simulink model "Alpha_Drone_Model"  (R2020b)
settings: Solver=VariableStepAuto  StartTime=0.0  StopTime=5  RelTol=1e-3
model workspace (MATLAB code in the model file):
  | % -------------------------------------------------------------------
  | %  Generated by MATLAB on 1-Mar-2021 14:46:59
  | %  MATLAB version: 9.9.0.1495850 (R2020b) Update 1
  | % -------------------------------------------------------------------
  | 
  | 
  | smiData = struct;
  | smiData.RigidTransform = struct;
  | smiData.RigidTransform(1).translation = ...
  |   [0 0 0];
  | smiData.RigidTransform(1).angle = 3.1415926535897931;
  | smiData.RigidTransform(1).axis = [1 0 0];
  | smiData.RigidTransform(1).ID = ['B[drone_base_test_3-1:-:drone_camera_w' ...
  |                                 'all_test-1]'];
  | smiData.RigidTransform(2).translation = ...
  |   [88.000000000000028 19.999999999999986 6.00000000000003];
  | smiData.RigidTransform(2).angle = 2.0943951023931953;
  | smiData.RigidTransform(2).axis = [0.57735026918962584 0.57735026918962584 ...
  |                                   -0.57735026918962562];
  | smiData.RigidTransform(2).ID = ['F[drone_base_test_3-1:-:drone_camera_w' ...
  |                                 'all_test-1]'];
  | smiData.RigidTransform(3).translation = ...
  |   [0 0 0];
  | smiData.RigidTransform(3).angle = 3.1415926535897931;
  | smiData.RigidTransform(3).axis = [1 0 0];
  | smiData.RigidTransform(3).ID = ['B[drone_base_test_3-1:-:drone_camera_w' ...
  |                                 'all_test-2]'];
  | smiData.RigidTransform(4).translation = ...
  |   [87.999999999999858 19.999999999999854 26.999999999999904];
  | smiData.RigidTransform(4).angle = 2.0943951023931953;
  | smiData.RigidTransform(4).axis = [0.57735026918962373 0.57735026918962573 ...
  |                                   -0.57735026918962784];
  | smiData.RigidTransform(4).ID = ['F[drone_base_test_3-1:-:drone_camera_w' ...
  |                                 'all_test-2]'];
  | smiData.RigidTransform(5).translation = ...
  |   [30.733125881400653 59.62221317792671 4.0000000000000036];
  | smiData.RigidTransform(5).angle = 3.1415926535897931;
  | smiData.RigidTransform(5).axis = [1 0 0];
  | smiData.RigidTransform(5).ID = ['B[drone_base_test_3-1:-:drone_top_test' ...
  |                                 '_3-1]'];
  | smiData.RigidTransform(6).translation = ...
  |   [30.733125881400646 59.622213177926717 26.999999999999986];
  | smiData.RigidTransform(6).angle = 3.1415926535897931;
  | smiData.RigidTransform(6).axis = [-1 -2.2204460492503131E-16 -0];
  | smiData.RigidTransform(6).ID = ['F[drone_base_test_3-1:-:drone_top_test' ...
  |                                 '_3-1]'];
  | smiData.RigidTransform(7).translation = ...
  |   [15 23.999999999999993 -1.0000000000000009];
  | smiData.RigidTransform(7).angle = 0;
  | smiData.RigidTransform(7).axis = [0 0 0];
  | smiData.RigidTransform(7).ID = ['B[drone_base_test_3-1:-:drone_fc_test-' ...
  |                                 '1]'];
  | smiData.RigidTransform(8).translation = ...
  |   [2.9999999999995808 29.999999999998998 2];
  | smiData.RigidTransform(8).angle = 2.3561944901923364;
  | smiData.RigidTransform(8).axis = [-0 -0 -1];
  | smiData.RigidTransform(8).ID = ['F[drone_base_test_3-1:-:drone_fc_test-' ...
  |                                 '1]'];
  | smiData.RigidTransform(9).translation = ...
  |   [0 0 4.0000000000000036];
  | smiData.RigidTransform(9).angle = 0;
  | smiData.RigidTransform(9).axis = [0 0 0];
  | smiData.RigidTransform(9).ID = ['B[drone_base_test_3-1:-:drone_arm_sing' ...
  |                                 'le_test_2_tl_br-2]'];
  | smiData.RigidTransform(10).translation = ...
  |   [17.677669529663881 38.890872965260449 3.9999999999995044];
  | smiData.RigidTransform(10).angle = 3.1415926535897869;
  | smiData.RigidTransform(10).axis = [0.92387953251128652 -0.38268343236509061 ...
  |                                    1.3170782690383521E-15];
  | smiData.RigidTransform(10).ID = ['F[drone_base_test_3-1:-:drone_arm_sin' ...
  |                                  'gle_test_2_tl_br-2]'];
  | smiData.RigidTransform(11).translation = ...
  |   [0 0 4.0000000000000036];
  | smiData.RigidTransform(11).angle = 0;
  | smiData.RigidTransform(11).axis = [0 0 0];
  | smiData.RigidTransform(11).ID = ['B[drone_base_test_3-1:-:drone_arm_sin' ...
  |                                  'gle_test_2_tl_br-3]'];
  | smiData.RigidTransform(12).translation = ...
  |   [-17.677669529664406 -38.890872965258076 4.0000000000005222];
  | smiData.RigidTransform(12).angle = 3.1415926535897905;
  | smiData.RigidTransform(12).axis = [0.38268343236509372 0.92387953251128518 ...
  |                                    -3.1797082198192578E-15];
  | smiData.RigidTransform(12).ID = ['F[drone_base_test_3-1:-:drone_arm_sin' ...
  |                                  'gle_test_2_tl_br-3]'];
  | smiData.RigidTransform(13).translation = ...
  |   [0 0 4.0000000000000036];
  | smiData.RigidTransform(13).angle = 0;
  | smiData.RigidTransform(13).axis = [0 0 0];
  | smiData.RigidTransform(13).ID = ['B[drone_base_test_3-1:-:drone_arm_sin' ...
  |                                  'gle_test_2_tr_bl-1]'];
  | smiData.RigidTransform(14).translation = ...
  |   [38.890872965259732 17.677669529664023 0];
  | smiData.RigidTransform(14).angle = 2.35619449019235;
  | smiData.RigidTransform(14).axis = [0 0 1];
  | smiData.RigidTransform(14).ID = ['F[drone_base_test_3-1:-:drone_arm_sin' ...
  |                                  'gle_test_2_tr_bl-1]'];
  | smiData.RigidTransform(15).translation = ...
  |   [0 0 4.0000000000000036];
  | smiData.RigidTransform(15).angle = 0;
  | smiData.RigidTransform(15).axis = [0 0 0];
  | smiData.RigidTransform(15).ID = ['B[drone_base_test_3-1:-:drone_arm_sin' ...
  |                                  'gle_test_2_tr_bl-2]'];
  | smiData.RigidTransform(16).translation = ...
  |   [-38.890872965260584 -17.67766952966349 0];
  | smiData.RigidTransform(16).angle = 0.78539816339744983;
  | smiData.RigidTransform(16).axis = [-0 -0 -1];
  | smiData.RigidTransform(16).ID = ['F[drone_base_test_3-1:-:drone_arm_sin' ...
  |                                  'gle_test_2_tr_bl-2]'];
  | smiData.RigidTransform(17).translation = ...
  |   [0 0 0];
  | smiData.RigidTransform(17).angle = 2.0943951023931953;
  | smiData.RigidTransform(17).axis = [-0.57735026918962584 -0.57735026918962584 ...
  |                                    -0.57735026918962584];
  | smiData.RigidTransform(17).ID = ['B[drone_camera_wall_test-1:-:drone_ca' ...
  |                                  'mera_and_proximity_sensor_weight-1]'];
  | smiData.RigidTransform(18).translation = ...
  |   [17.9999999999999 15.000000000000691 -1.8349766151004587E-12];
  | smiData.RigidTransform(18).angle = 1.5707963267948863;
  | smiData.RigidTransform(18).axis = [1 -7.1439206870112137E-15 3.5419578862734405E-15 ...
  |                                    ];
  | smiData.RigidTransform(18).ID = ['F[drone_camera_wall_test-1:-:drone_ca' ...
  |                                  'mera_and_proximity_sensor_weight-1]'];
  | smiData.RigidTransform(19).translation = ...
  |   [0 0 0];
  | smiData.RigidTransform(19).angle = 3.1415926535897931;
  | smiData.RigidTransform(19).axis = [1 0 0];
  | smiData.RigidTransform(19).ID = ['B[drone_top_test_3-1:-:drone_battery_' ...
  |                                  'cell_1-1]'];
  | smiData.RigidTransform(20).translation = ...
  |   [28.499999999996163 13.499999999999471 7.4000000000009329];
  | smiData.RigidTransform(20).angle = 3.1415926535897838;
  | smiData.RigidTransform(20).axis = [2.3314683517128287E-15 -0.70710678118654646 ...
  |                                    0.70710678118654879];
  | smiData.RigidTransform(20).ID = ['F[drone_top_test_3-1:-:drone_battery_' ...
  |                                  'cell_1-1]'];
  | smiData.RigidTransform(21).translation = ...
  |   [0 0 11.300000000000004];
  | smiData.RigidTransform(21).angle = 3.1415926535897931;
  | smiData.RigidTransform(21).axis = [1 0 0];
  | smiData.RigidTransform(21).ID = ['B[drone_motor_test_3-2:-:drone_propel' ...
  |                                  'ler_2_tl_br-3]'];
  | smiData.RigidTransform(22).translation = ...
  |   [-1.0691831202990747E-12 -9.0949470177292824E-13 1.4999999999994174];
  | smiData.RigidTransform(22).angle = 3.1415926535897865;
  | smiData.RigidTransform(22).axis = [-1 1.2016601214541445E-29 -3.4914813388431452E-15 ...
  |                                    ];
  | smiData.RigidTransform(22).ID = ['F[drone_motor_test_3-2:-:drone_propel' ...
  |                                  'ler_2_tl_br-3]'];
  | smiData.RigidTransform(23).translation = ...
  |   [4.2426406871192288 99.242640687119334 3.99999999999999];
  | smiData.RigidTransform(23).angle = 3.1415926535897931;
  | smiData.RigidTransform(23).axis = [1 0 0];
  | smiData.RigidTransform(23).ID = ['B[drone_arm_single_test_2_tl_br-3:-:d' ...
  |                                  'rone_motor_test_3-2]'];
  | smiData.RigidTransform(24).translation = ...
  |   [-5.9999999999979607 1.6080470288670991E-12 -3.9999999999987779];
  | smiData.RigidTransform(24).angle = 3.1415926535897931;
  | smiData.RigidTransform(24).axis = [0.38268343236508745 0.92387953251128774 ...
  |                                    -6.3594164396385283E-15];
  | smiData.RigidTransform(24).ID = ['F[drone_arm_single_test_2_tl_br-3:-:d' ...
  |                                  'rone_motor_test_3-2]'];
  | smiData.RigidTransform(25).translation = ...
  |   [0 0 11.300000000000004];
  | smiData.RigidTransform(25).angle = 3.1415926535897931;
  | smiData.RigidTransform(25).axis = [1 0 0];
  | smiData.RigidTransform(25).ID = ['B[drone_motor_test_3-3:-:drone_propel' ...
  |                                  'ler_2_tl_br-4]'];
  | smiData.RigidTransform(26).translation = ...
  |   [-1.630511881549574E-12 -4.6895820560166612E-13 1.5000000000023306];
  | smiData.RigidTransform(26).angle = 3.1415926535897931;
  | smiData.RigidTransform(26).axis = [1 8.2125091513898182E-44 6.9331727151811155E-15 ...
  |                                    ];
  | smiData.RigidTransform(26).ID = ['F[drone_motor_test_3-3:-:drone_propel' ...
  |                                  'ler_2_tl_br-4]'];
  | smiData.RigidTransform(27).translation = ...
  |   [0 0 4.0000000000000036];
  | smiData.RigidTransform(27).angle = 0;
  | smiData.RigidTransform(27).axis = [0 0 0];
  | smiData.RigidTransform(27).ID = ['B[drone_arm_single_test_2_tl_br-2:-:d' ...
  |                                  'rone_motor_test_3-3]'];
  | smiData.RigidTransform(28).translation = ...
  |   [67.175144212722017 67.1751442127213 -4.0000000000004334];
  | smiData.RigidTransform(28).angle = 2.3561944901923431;
  | smiData.RigidTransform(28).axis = [-2.0160961307562574E-15 2.0160961307562506E-15 ...
  |                                    1];
  | smiData.RigidTransform(28).ID = ['F[drone_arm_single_test_2_tl_br-2:-:d' ...
  |                                  'rone_motor_test_3-3]'];
  | smiData.RigidTransform(29).translation = ...
  |   [0 0 11.300000000000004];
  | smiData.RigidTransform(29).angle = 3.1415926535897931;
  | smiData.RigidTransform(29).axis = [1 0 0];
  | smiData.RigidTransform(29).ID = ['B[drone_motor_test_3-4:-:drone_propel' ...
  |                                  'ler_2_tr_bl-1]'];
  | smiData.RigidTransform(30).translation = ...
  |   [-2.6469353547492776E-16 -3.542839513132647E-15 -1.4999999999999574];
  | smiData.RigidTransform(30).angle = 1.0594127220296946E-16;
  | smiData.RigidTransform(30).axis = [-0.074504606733252654 -0.99722066944860466 ...
  |                                    3.9355876263450373E-18];
  | smiData.RigidTransform(30).ID = ['F[drone_motor_test_3-4:-:drone_propel' ...
  |                                  'ler_2_tr_bl-1]'];
  | smiData.RigidTransform(31).translation = ...
  |   [0 0 0];
  | smiData.RigidTransform(31).angle = 3.1415926535897931;
  | smiData.RigidTransform(31).axis = [1 0 0];
  | smiData.RigidTransform(31).ID = ['B[drone_arm_single_test_2_tr_bl-2:-:d' ...
  |                                  'rone_motor_test_3-4]'];
  | smiData.RigidTransform(32).translation = ...
  |   [67.175144212721548 67.175144212722486 -4.0000000000000071];
  | smiData.RigidTransform(32).angle = 0.78539816339744117;
  | smiData.RigidTransform(32).axis = [-1.278824280837353E-16 -5.2970636101485407E-17 ...
  |                                    -1];
  | smiData.RigidTransform(32).ID = ['F[drone_arm_single_test_2_tr_bl-2:-:d' ...
  |                                  'rone_motor_test_3-4]'];
  | smiData.RigidTransform(33).translation = ...
  |   [0 0 11.300000000000004];
  | smiData.RigidTransform(33).angle = 3.1415926535897931;
  | smiData.RigidTransform(33).axis = [1 0 0];
  | smiData.RigidTransform(33).ID = ['B[drone_motor_test_3-5:-:drone_propel' ...
  |                                  'ler_2_tr_bl-2]'];
  | smiData.RigidTransform(34).translation = ...
  |   [-5.6843418860808015E-14 0 -1.5];
  | smiData.RigidTransform(34).angle = 1.1879803848348683E-16;
  | smiData.RigidTransform(34).axis = [1 4.8038803367965795E-14 2.8534578056041286E-30 ...
  |                                    ];
  | smiData.RigidTransform(34).ID = ['F[drone_motor_test_3-5:-:drone_propel' ...
  |                                  'ler_2_tr_bl-2]'];
  | smiData.RigidTransform(35).translation = ...
  |   [0 0 0];
  | smiData.RigidTransform(35).angle = 3.1415926535897931;
  | smiData.RigidTransform(35).axis = [1 0 0];
  | smiData.RigidTransform(35).ID = ['B[drone_arm_single_test_2_tr_bl-1:-:d' ...
  |                                  'rone_motor_test_3-5]'];
  | smiData.RigidTransform(36).translation = ...
  |   [67.175144212721165 67.175144212722813 -4.0000000000000071];
  | smiData.RigidTransform(36).angle = 0.78539816339743962;
  | smiData.RigidTransform(36).axis = [5.9399019241738509E-17 -1.4340191784508119E-16 ...
  |                                    -1];
  | smiData.RigidTransform(36).ID = ['F[drone_arm_single_test_2_tr_bl-1:-:d' ...
  |                                  'rone_motor_test_3-5]'];
  | smiData.RigidTransform(37).translation = ...
  |   [0 2.2679491924310624 3.33974596215561];
  | smiData.RigidTransform(37).angle = 0.52359877559829271;
  | smiData.RigidTransform(37).axis = [1 0 0];
  | smiData.RigidTransform(37).ID = ['B[drone_antenna_holder_test-1:-:drone' ...
  |                                  '_antenna_test-1]'];
  | smiData.RigidTransform(38).translation = ...
  |   [-7.1054273576010019E-14 2.1316282072803006E-14 -60.000000000000043];
  | smiData.RigidTransform(38).angle = 2.2887833992611192E-16;
  | smiData.RigidTransform(38).axis = [0.9552871077824594 -0.29567979590195814 ...
  |                                    -3.2324384615704697E-17];
  | smiData.RigidTransform(38).ID = ['F[drone_antenna_holder_test-1:-:drone' ...
  |                                  '_antenna_test-1]'];
  | smiData.RigidTransform(39).translation = ...
  |   [0 0 4.0000000000000036];
  | smiData.RigidTransform(39).angle = 0;
  | smiData.RigidTransform(39).axis = [0 0 0];
  | smiData.RigidTransform(39).ID = ['B[drone_arm_single_test_2_tl_br-2:-:d' ...
  |                                  'rone_esc_1_1_test-4]'];
  | smiData.RigidTransform(40).translation = ...
  |   [-44.500000000001137 6.0000000000001705 2.4999999999997442];
  | smiData.RigidTransform(40).angle = 3.1415926535897882;
  | smiData.RigidTransform(40).axis = [-0.70710678118654624 -0.70710678118654891 ...
  |                                    2.433643310959854E-15];
  | smiData.RigidTransform(40).ID = ['F[drone_arm_single_test_2_tl_br-2:-:d' ...
  |                                  'rone_esc_1_1_test-4]'];
  | smiData.RigidTransform(41).translation = ...
  |   [0 0 4.0000000000000036];
  | smiData.RigidTransform(41).angle = 0;
  | smiData.RigidTransform(41).axis = [0 0 0];
  | smiData.RigidTransform(41).ID = ['B[drone_arm_single_test_2_tl_br-3:-:d' ...
  |                                  'rone_esc_1_1_test-1]'];
  | smiData.RigidTransform(42).translation = ...
  |   [68.000000000001648 6 2.5000000000002558];
  | smiData.RigidTransform(42).angle = 3.1415926535897882;
  | smiData.RigidTransform(42).axis = [-0.70710678118654646 0.70710678118654879 ...
  |                                    -2.4336433109598548E-15];
  | smiData.RigidTransform(42).ID = ['F[drone_arm_single_test_2_tl_br-3:-:d' ...
  |                                  'rone_esc_1_1_test-1]'];
  | smiData.RigidTransform(43).translation = ...
  |   [0 0 0];
  | smiData.RigidTransform(43).angle = 3.1415926535897931;
  | smiData.RigidTransform(43).axis = [1 0 0];
  | smiData.RigidTransform(43).ID = ['B[drone_arm_single_test_2_tr_bl-1:-:d' ...
  |                                  'rone_esc_1_1_test-3]'];
  | smiData.RigidTransform(44).translation = ...
  |   [-44.500000000000085 5.9999999999999716 2.4999999999999858];
  | smiData.RigidTransform(44).angle = 3.1415926535897931;
  | smiData.RigidTransform(44).axis = [-0.70710678118654757 0.70710678118654757 ...
  |                                    0];
  | smiData.RigidTransform(44).ID = ['F[drone_arm_single_test_2_tr_bl-1:-:d' ...
  |                                  'rone_esc_1_1_test-3]'];
  | smiData.RigidTransform(45).translation = ...
  |   [0 0 0];
  | smiData.RigidTransform(45).angle = 3.1415926535897931;
  | smiData.RigidTransform(45).axis = [1 0 0];
  | smiData.RigidTransform(45).ID = ['B[drone_arm_single_test_2_tr_bl-2:-:d' ...
  |                                  'rone_esc_1_1_test-2]'];
  | smiData.RigidTransform(46).translation = ...
  |   [-44.500000000000163 5.9999999999998614 2.5];
  | smiData.RigidTransform(46).angle = 3.1415926535897931;
  | smiData.RigidTransform(46).axis = [-0.70710678118654746 0.70710678118654757 ...
  |                                    0];
  | smiData.RigidTransform(46).ID = ['F[drone_arm_single_test_2_tr_bl-2:-:d' ...
  |                                  'rone_esc_1_1_test-2]'];
  | smiData.RigidTransform(47).translation = ...
  |   [25 14.999999999999986 -1.0000000000000009];
  | smiData.RigidTransform(47).angle = 0;
  | smiData.RigidTransform(47).axis = [0 0 0];
  | smiData.RigidTransform(47).ID = ['B[drone_base_test_3-1:-:drone_chip_2_' ...
  |                                  'test-1]'];
  | smiData.RigidTransform(48).translation = ...
  |   [10.000000000000682 -10.00000000000145 2];
  | smiData.RigidTransform(48).angle = 1.5707963267948861;
  | smiData.RigidTransform(48).axis = [-0 -0 -1];
  | smiData.RigidTransform(48).ID = ['F[drone_base_test_3-1:-:drone_chip_2_' ...
  |                                  'test-1]'];
  | smiData.RigidTransform(49).translation = ...
  |   [13.499999999999998 -13.499999999999984 69.999999999999986];
  | smiData.RigidTransform(49).angle = 2.0943951023931953;
  | smiData.RigidTransform(49).axis = [0.57735026918962584 0.57735026918962584 ...
  |                                    0.57735026918962584];
  | smiData.RigidTransform(49).ID = ['B[drone_battery_cell_1-1:-:drone_batt' ...
  |                                  'ery_cell_1-2]'];
  | smiData.RigidTransform(50).translation = ...
  |   [-13.500000000000014 -13.500000000000313 69.999999999999915];
  | smiData.RigidTransform(50).angle = 2.0943951023931957;
  | smiData.RigidTransform(50).axis = [0.577350269189626 0.57735026918962573 ...
  |                                    0.57735026918962562];
  | smiData.RigidTransform(50).ID = ['F[drone_battery_cell_1-1:-:drone_batt' ...
  |                                  'ery_cell_1-2]'];
  | smiData.RigidTransform(51).translation = ...
  |   [0 0 0];
  | smiData.RigidTransform(51).angle = 3.1415926535897931;
  | smiData.RigidTransform(51).axis = [1 0 0];
  | smiData.RigidTransform(51).ID = ['B[drone_base_test_3-1:-:drone_antenna' ...
  |                                  '_holder_test-1]'];
  | smiData.RigidTransform(52).translation = ...
  |   [15.000000000000412 9.99999999999984 1.7725906433550571E-15];
  | smiData.RigidTransform(52).angle = 3.1415926535897918;
  | smiData.RigidTransform(52).axis = [5.9086354778499992E-17 4.0675640425458421E-31 ...
  |                                    -1];
  | smiData.RigidTransform(52).ID = ['F[drone_base_test_3-1:-:drone_antenna' ...
  |                                  '_holder_test-1]'];
  | smiData.RigidTransform(53).translation = ...
  |   [30.733125881400653 59.62221317792671 4.0000000000000036];
  | smiData.RigidTransform(53).angle = 3.1415926535897931;
  | smiData.RigidTransform(53).axis = [1 0 0];
  | smiData.RigidTransform(53).ID = ['B[drone_base_test_3-1:-:drone_pillar_' ...
  |                                  'test_2-1]'];
  | smiData.RigidTransform(54).translation = ...
  |   [0 0 23.999999999999986];
  | smiData.RigidTransform(54).angle = 3.1415926535897931;
  | smiData.RigidTransform(54).axis = [1 0 0];
  | smiData.RigidTransform(54).ID = ['F[drone_base_test_3-1:-:drone_pillar_' ...
  |                                  'test_2-1]'];
  | smiData.RigidTransform(55).translation = ...
  |   [0 0 0];
  | smiData.RigidTransform(55).angle = 3.1415926535897931;
  | smiData.RigidTransform(55).axis = [1 0 0];
  | smiData.RigidTransform(55).ID = ['B[drone_pillar_test_2-1:-:drone_top_t' ...
  |                                  'est_3-1]'];
  | smiData.RigidTransform(56).translation = ...
  |   [30.733125881400646 59.622213177926717 3];
  | smiData.RigidTransform(56).angle = 3.1415926535897931;
  | smiData.RigidTransform(56).axis = [1 0 0];
  | smiData.RigidTransform(56).ID = ['F[drone_pillar_test_2-1:-:drone_top_t' ...
  |                                  'est_3-1]'];
  | smiData.RigidTransform(57).translation = ...
  |   [-0.733125881400648 59.62221317792671 4.0000000000000036];
  | smiData.RigidTransform(57).angle = 3.1415926535897931;
  | smiData.RigidTransform(57).axis = [1 0 0];
  | smiData.RigidTransform(57).ID = ['B[drone_base_test_3-1:-:drone_pillar_' ...
  |                                  'test_2-2]'];
  | smiData.RigidTransform(58).translation = ...
  |   [-1.4210854715202004E-14 7.1054273576010019E-15 23.999999999999986];
  | smiData.RigidTransform(58).angle = 3.1415926535897931;
  | smiData.RigidTransform(58).axis = [1 0 0];
  | smiData.RigidTransform(58).ID = ['F[drone_base_test_3-1:-:drone_pillar_' ...
  |                                  'test_2-2]'];
  | smiData.RigidTransform(59).translation = ...
  |   [30.733125881400653 20.377786822073265 4.0000000000000036];
  | smiData.RigidTransform(59).angle = 3.1415926535897931;
  | smiData.RigidTransform(59).axis = [1 0 0];
  | smiData.RigidTransform(59).ID = ['B[drone_base_test_3-1:-:drone_pillar_' ...
  |                                  'test_2-3]'];
  | smiData.RigidTransform(60).translation = ...
  |   [1.0091756082984115E-13 -5.2348285428429971E-14 24.000000000000014];
  | smiData.RigidTransform(60).angle = 3.1415926535897931;
  | smiData.RigidTransform(60).axis = [1 0 0];
  | smiData.RigidTransform(60).ID = ['F[drone_base_test_3-1:-:drone_pillar_' ...
  |                                  'test_2-3]'];
  | smiData.RigidTransform(61).translation = ...
  |   [-0.733125881400648 20.377786822073279 4.0000000000000036];
  | smiData.RigidTransform(61).angle = 3.1415926535897931;
  | smiData.RigidTransform(61).axis = [1 0 0];
  | smiData.RigidTransform(61).ID = ['B[drone_base_test_3-1:-:drone_pillar_' ...
  |                                  'test_2-4]'];
  | smiData.RigidTransform(62).translation = ...
  |   [-2.8421709430404007E-14 -7.1054273576010019E-15 23.999999999999986];
  | smiData.RigidTransform(62).angle = 3.1415926535897931;
  | smiData.RigidTransform(62).axis = [1 0 0];
  | smiData.RigidTransform(62).ID = ['F[drone_base_test_3-1:-:drone_pillar_' ...
  |                                  'test_2-4]'];
  | smiData.RigidTransform(63).translation = ...
  |   [-141.02635015453362 -35.750624234736684 -110.79224989420835];
  | smiData.RigidTransform(63).angle = 1.5707963267948861;
  | smiData.RigidTransform(63).axis = [0 0 -1];
  | smiData.RigidTransform(63).ID = 'RootGround[drone_base_test_3-1]';
  | smiData.Solid = struct;
  | smiData.Solid(1).mass = 0.0013591771119401339;
  | smiData.Solid(1).CoM = [6.2782672784602285E-9 -3.005481690319291E-10 -0.13654023366223458 ...
  |                         ];
  | smiData.Solid(1).MoI = [0.0066878929643460752 0.83698629203444719 0.84230803636261442 ...
  |                         ];
  | smiData.Solid(1).PoI = [0 0 -0.012369136319665996];
  | smiData.Solid(1).color = [1 1 1];
  | smiData.Solid(1).opacity = 1;
  | smiData.Solid(1).ID = 'drone_propeller_2_tl_br*:*Défaut';
  | smiData.Solid(2).mass = 0.04;
  | smiData.Solid(2).CoM = [9 4.9999999999999991 4.7862823653085078];
  | smiData.Solid(2).MoI = [0.69557200020051613 1.4099541203730128 1.3591823458658341 ...
  |                         ];
  | smiData.Solid(2).PoI = [0 0 -5.2310768304219234E-7];
  | smiData.Solid(2).color = [0.792156862745098 0.81960784313725488 0.93333333333333335 ...
  |                           ];
  | smiData.Solid(2).opacity = 1;
  | smiData.Solid(2).ID = ['drone_camera_and_proximity_sensor_weight*:*Défa' ...
  |                        'ut'];
  | smiData.Solid(3).mass = 0.0068469637400900823;
  | smiData.Solid(3).CoM = [-0.11657640817340231 61.037498975827987 2.1074901885463913 ...
  |                         ];
  | smiData.Solid(3).MoI = [4.6018431505699775 0.15800553957661936 4.7423288035223932 ...
  |                         ];
  | smiData.Solid(3).PoI = [0.003685148800022439 0.00038191256844076656 -0.044289576986049982 ...
  |                         ];
  | smiData.Solid(3).color = [1 1 1];
  | smiData.Solid(3).opacity = 1;
  | smiData.Solid(3).ID = 'drone_arm_single_test_2_tl_br*:*Défaut';
  | smiData.Solid(4).mass = 0.00037472917172019045;
  | smiData.Solid(4).CoM = [0 0 9.9999999999999982];
  | smiData.Solid(4).MoI = [0.013364091360781051 0.013364091360781051 0.0017462379402160874 ...
  |                         ];
  | smiData.Solid(4).PoI = [0 0 0];
  | smiData.Solid(4).color = [1 1 1];
  | smiData.Solid(4).opacity = 1;
  | smiData.Solid(4).ID = 'drone_pillar_test_2*:*Défaut';
  | smiData.Solid(5).mass = 0.032799999999999996;
  | smiData.Solid(5).CoM = [0 0 -3.8314295222245094];
  | smiData.Solid(5).MoI = [8.7908062706846515 8.7908062706846515 0.64055397546142256 ...
  |                         ];
  | smiData.Solid(5).PoI = [0 0 0];
  | smiData.Solid(5).color = [0.792156862745098 0.81960784313725488 0.93333333333333335 ...
  |                           ];
  | smiData.Solid(5).opacity = 1;
  | smiData.Solid(5).ID = 'drone_antenna_test*:*Défaut';
  | smiData.Solid(6).mass = 0.00094110152190793133;
  | smiData.Solid(6).CoM = [2.037067460789641E-6 -0.49634576864971031 10.419198342323027 ...
  |                         ];
  | smiData.Solid(6).MoI = [0.033392915764434816 0.050182738401604074 0.024962462698705997 ...
  |                         ];
  | smiData.Solid(6).PoI = [0.00258495880062068 -1.1200684489948608E-8 2.9162151030672723E-9 ...
  |                         ];
  | smiData.Solid(6).color = [1 1 1];
  | smiData.Solid(6).opacity = 1;
  | smiData.Solid(6).ID = 'drone_antenna_holder_test*:*Défaut';
  | smiData.Solid(7).mass = 0.00229211560497973;
  | smiData.Solid(7).CoM = [13.09867757647158 10.15947919220863 1.4999999999999998 ...
  |                         ];
  | smiData.Solid(7).MoI = [0.098259458477035683 0.12375362309991163 0.21863889652134511 ...
  |                         ];
  | smiData.Solid(7).PoI = [0 0 -0.0030710592640717372];
  | smiData.Solid(7).color = [1 1 1];
  | smiData.Solid(7).opacity = 1;
  | smiData.Solid(7).ID = 'drone_camera_wall_test*:*Défaut';
  | smiData.Solid(8).mass = 0.015266276862112403;
  | smiData.Solid(8).CoM = [15.000000000000002 30.413343580259017 2];
  | smiData.Solid(8).MoI = [7.9686336012081416 1.7172121717776689 9.64513570135351 ...
  |                         ];
  | smiData.Solid(8).PoI = [0 0 0];
  | smiData.Solid(8).color = [1 1 1];
  | smiData.Solid(8).opacity = 1;
  | smiData.Solid(8).ID = 'drone_base_test_3*:*Défaut';
  | smiData.Solid(9).mass = 0.015;
  | smiData.Solid(9).CoM = [16.5 16.500000000000004 1.5];
  | smiData.Solid(9).MoI = [1.3174433817628703 1.3174433817628706 2.6125367080637742 ...
  |                         ];
  | smiData.Solid(9).PoI = [0 0 0];
  | smiData.Solid(9).color = [0.792156862745098 0.81960784313725488 0.93333333333333335 ...
  |                           ];
  | smiData.Solid(9).opacity = 1;
  | smiData.Solid(9).ID = 'drone_fc_test*:*Défaut';
  | smiData.Solid(10).mass = 0.06;
  | smiData.Solid(10).CoM = [0 0 35.000000000000014];
  | smiData.Solid(10).MoI = [28.098928197297447 28.098928197297447 7.2838974183990253 ...
  |                          ];
  | smiData.Solid(10).PoI = [0 0 0];
  | smiData.Solid(10).color = [0.792156862745098 0.81960784313725488 0.93333333333333335 ...
  |                            ];
  | smiData.Solid(10).opacity = 1;
  | smiData.Solid(10).ID = 'drone_battery_cell_1*:*Défaut';
  | smiData.Solid(11).mass = 0.011175377260713786;
  | smiData.Solid(11).CoM = [15.000000000000002 29.323067981096848 1.5000000000000002 ...
  |                          ];
  | smiData.Solid(11).MoI = [6.0401869060719253 1.0425872200991047 7.0660110602799575 ...
  |                          ];
  | smiData.Solid(11).PoI = [0 0 0];
  | smiData.Solid(11).color = [1 1 1];
  | smiData.Solid(11).opacity = 1;
  | smiData.Solid(11).ID = 'drone_top_test_3*:*Défaut';
  | smiData.Solid(12).mass = 0.01;
  | smiData.Solid(12).CoM = [0 0 1.5000000000000002];
  | smiData.Solid(12).MoI = [0.53835367084795227 0.53835367084795238 1.0618343791423916 ...
  |                          ];
  | smiData.Solid(12).PoI = [0 0 0];
  | smiData.Solid(12).color = [0.792156862745098 0.81960784313725488 0.93333333333333335 ...
  |                            ];
  | smiData.Solid(12).opacity = 1;
  | smiData.Solid(12).ID = 'drone_chip_2_test*:*Défaut';
  | smiData.Solid(13).mass = 0.0068469630253905588;
  | smiData.Solid(13).CoM = [-0.11656686315053104 61.037502482876086 1.8925100183584762 ...
  |                          ];
  | smiData.Solid(13).MoI = [4.6018422965837562 0.15800552901932971 4.7423279440874309 ...
  |                          ];
  | smiData.Solid(13).PoI = [-0.0036850978277272965 -0.00038177097939288626 ...
  |                          -0.044289044671629446];
  | smiData.Solid(13).color = [1 1 1];
  | smiData.Solid(13).opacity = 1;
  | smiData.Solid(13).ID = 'drone_arm_single_test_2_tr_bl*:*Défaut';
  | smiData.Solid(14).mass = 0.01;
  | smiData.Solid(14).CoM = [0.31851522822486505 0.31851530348302387 2.5290314994017158 ...
  |                          ];
  | smiData.Solid(14).MoI = [0.30076847891404196 0.29810667222008319 0.40106404927730616 ...
  |                          ];
  | smiData.Solid(14).PoI = [0.01124048760894434 0.011240491544358239 -0.022721274336399915 ...
  |                          ];
  | smiData.Solid(14).color = [0.68627450980392157 0.6588235294117647 0.63921568627450975 ...
  |                            ];
  | smiData.Solid(14).opacity = 1;
  | smiData.Solid(14).ID = 'drone_motor_test_3*:*Défaut';
  | smiData.Solid(15).mass = 0.0045000000000000005;
  | smiData.Solid(15).CoM = [11.75 6 1.25];
  | smiData.Solid(15).MoI = [0.056343750000000019 0.2094375 0.26109375];
  | smiData.Solid(15).PoI = [0 0 0];
  | smiData.Solid(15).color = [0.792156862745098 0.81960784313725488 0.93333333333333335 ...
  |                            ];
  | smiData.Solid(15).opacity = 1;
  | smiData.Solid(15).ID = 'drone_esc_1_1_test*:*Défaut';
  | smiData.Solid(16).mass = 0.0013591765923234771;
  | smiData.Solid(16).CoM = [1.1950397153793501E-9 -2.9281418394781323E-11 ...
  |                          0.13654053545657041];
  | smiData.Solid(16).MoI = [0.006687902009900896 0.83697880572861283 0.84230057195809283 ...
  |                          ];
  | smiData.Solid(16).PoI = [0 0 -0.012369029069616478];
  | smiData.Solid(16).color = [1 1 1];
  | smiData.Solid(16).opacity = 1;
  | smiData.Solid(16).ID = 'drone_propeller_2_tr_bl*:*Défaut';
  | smiData.PlanarJoint = struct;
  | smiData.PlanarJoint.Rz = struct;
  | smiData.PlanarJoint.Rz.Pos = -154.16759191545947;
  | smiData.PlanarJoint.Px = struct;
  | smiData.PlanarJoint.Px.Pos = 0;
  | smiData.PlanarJoint.Py = struct;
  | smiData.PlanarJoint.Py.Pos = 0;
  | smiData.PlanarJoint.ID = '[drone_pillar_test_2-1:-:drone_top_test_3-1]';
  | smiData.PrismaticJoint = struct;
  | smiData.PrismaticJoint(1).Pz = struct;
  | smiData.PrismaticJoint(1).Pz.Pos = 0;
  | smiData.PrismaticJoint(1).ID = ['[drone_base_test_3-1:-:drone_top_test_' ...
  |                                 '3-1]'];
  | smiData.PrismaticJoint(2).Pz = struct;
  | smiData.PrismaticJoint(2).Pz.Pos = 0;
  | smiData.PrismaticJoint(2).ID = ['[drone_camera_wall_test-1:-:drone_came' ...
  |                                 'ra_and_proximity_sensor_weight-1]'];
  | smiData.RevoluteJoint = struct;
  | smiData.RevoluteJoint(1).Rz = struct;
  | smiData.RevoluteJoint(1).Rz.Pos = -3.9438878050147319E-13;
  | smiData.RevoluteJoint(1).ID = ['[drone_motor_test_3-2:-:drone_propeller' ...
  |                                '_2_tl_br-3]'];
  | smiData.RevoluteJoint(2).Rz = struct;
  | smiData.RevoluteJoint(2).Rz.Pos = 179.99999999999963;
  | smiData.RevoluteJoint(2).ID = ['[drone_motor_test_3-3:-:drone_propeller' ...
  |                                '_2_tl_br-4]'];
  | smiData.RevoluteJoint(3).Rz = struct;
  | smiData.RevoluteJoint(3).Rz.Pos = 94.272758723662335;
  | smiData.RevoluteJoint(3).ID = ['[drone_motor_test_3-4:-:drone_propeller' ...
  |                                '_2_tr_bl-1]'];
  | smiData.RevoluteJoint(4).Rz = struct;
  | smiData.RevoluteJoint(4).Rz.Pos = -90.0000000000008;
  | smiData.RevoluteJoint(4).ID = ['[drone_motor_test_3-5:-:drone_propeller' ...
  |                                '_2_tr_bl-2]'];
  | smiData.RevoluteJoint(5).Rz = struct;
  | smiData.RevoluteJoint(5).Rz.Pos = 6.3241238202382242;
  | smiData.RevoluteJoint(5).ID = ['[drone_antenna_holder_test-1:-:drone_an' ...
  |                                'tenna_test-1]'];
  | smiData.RevoluteJoint(6).Rz = struct;
  | smiData.RevoluteJoint(6).Rz.Pos = 154.1675919154595;
  | smiData.RevoluteJoint(6).ID = ['[drone_base_test_3-1:-:drone_pillar_tes' ...
  |                                't_2-1]'];
  | smiData.RevoluteJoint(7).Rz = struct;
  | smiData.RevoluteJoint(7).Rz.Pos = -89.9999999999994;
  | smiData.RevoluteJoint(7).ID = ['[drone_base_test_3-1:-:drone_pillar_tes' ...
  |                                't_2-2]'];
  | smiData.RevoluteJoint(8).Rz = struct;
  | smiData.RevoluteJoint(8).Rz.Pos = 62.583180499697804;
  | smiData.RevoluteJoint(8).ID = ['[drone_base_test_3-1:-:drone_pillar_tes' ...
  |                                't_2-3]'];
  | smiData.RevoluteJoint(9).Rz = struct;
  | smiData.RevoluteJoint(9).Rz.Pos = -89.9999999999994;
  | smiData.RevoluteJoint(9).ID = ['[drone_base_test_3-1:-:drone_pillar_tes' ...
  |                                't_2-4]'];
undefined symbols (not defined in the file or in its folder): g, R, V1_trim, V3_trim, X, Y, Z
libraries: sm_lib x149, fl_lib x113, nesl_utility x52, ee_lib x16
(part 1 of 5)
settings Model: Creator=jbmic  LastModifiedBy=maria
settings DataIOCC: ReturnWorkspaceOutputs=off

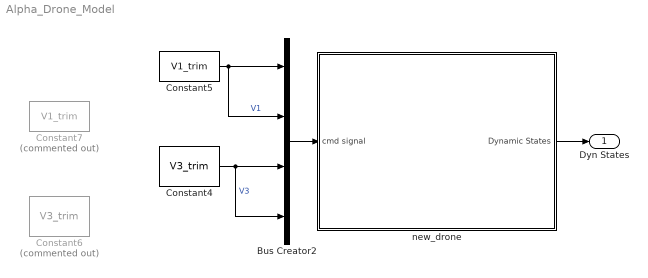
== system Alpha_Drone_Model ==
  Bus Creator2 : BusCreator  Inputs=4
  Constant4 : Constant  Value=V3_trim
  Constant5 : Constant  Value=V1_trim
  Constant6 : Constant  Commented=on  Value=V3_trim
  Constant7 : Constant  Commented=on  Value=V1_trim
  new_drone : Subsystem
  Dyn States : Outport
  wires:
  new_drone/1(Dynamic States) -> Dyn States/1
  Constant5/1 -> Bus Creator2/2, Bus Creator2/1  "V1"
  Bus Creator2/1 -> new_drone/1(cmd signal)
  Constant4/1 -> Bus Creator2/3, Bus Creator2/4  "V3"
